simulink model "FM_V6_Zikun"  (R2022b)
settings: Solver=VariableStepAuto  StartTime=0.0  StopTime=1240
values from neighbouring files (symbols this model uses):
  A_fc = 550    [CNV.m]
  A_st = 1.1*A_fc*1E-4*n_cell*0.0012    (= 0.047553)    [CNV.m]
  A_T_rm = 0.005    [CNV.m]
  b11 = 0.005139    [CNV.m]
  b12 = 0.00326    [CNV.m]
  b2 = 350    [CNV.m]
  c1 = 10    [CNV.m]
  c3 = 2    [CNV.m]
  cc = 30    [CNV.m]
  Cd_rm = 0.0124    [CNV.m]
  Cp_air = 1005    [CNV.m]
  Cp_cl = 4180    [CNV.m]
  Cp_st = Cp_Al*1.5    (= 1350)    [CNV.m]
  F = 96485    [CNV.m]
  gamma = 1.4    [CNV.m]
  H_conv_st = 3    [CNV.m]
  i_max = 2.2    [CNV.m]
  k_ca_out = 0.2177*10^(-5)    (= 2.177e-06)    [CNV.m]
  K_sm_out = 0.3629*10^-5    (= 3.629e-06)    [CNV.m]
  kd_cp = 0.01    [CNV.m]
  kd_rm = 0    [CNV.m]
  ki_cp = 0.1    [CNV.m]
  ki_fan = -1E-5    (= -1e-05)    [CNV.m]
  ki_rm = -5E-8    (= -5e-08)    [CNV.m]
  kp_cp = 7.5    [CNV.m]
  kp_fan = -0.5    [CNV.m]
  kp_rm = -8E-7    (= -8e-07)    [CNV.m]
  M_a = 29*10^-3    (= 0.029)    [CNV.m]
  M_H2 = 2*10^-3    (= 0.002)    [CNV.m]
  m_H2_initial = P_atm*V_an/(R_H2*T_atm)    (= 0.00044494386048)    [CNV.m]
  m_H2O_initial = 0.005    [CNV.m]
  M_m_dry = 1.1    [CNV.m]
  M_N2 = 28*10^-3    (= 0.028)    [CNV.m]
  m_N2_initial = P_atm*(1-y_O2)*V_ca/(R_N2*T_atm)    (= 0.00586138039643)    [CNV.m]
  M_O2 = 32*10^-3    (= 0.032)    [CNV.m]
  m_O2_initial = P_atm*y_O2*V_ca/(R_O2*T_atm)    (= 0.00177998712422)    [CNV.m]
  m_st = n_cell*A_fc*t_m*rho_m_dry+(V_ca+V_an)*rho_Al*2.5    (= 87.4506875)    [CNV.m]
  M_v = 18*10^-3    (= 0.018)    [CNV.m]
  n_cell = 655    [CNV.m]
  P_a = P_atm*(1-L*h/T_atm)^(g*M_a/(R*L))    [CNV.m]
  P_atm = 101.25*10^3    (= 101250)    [CNV.m]
  P_ca_ref = 2.5*P_a    [CNV.m]
  phi_a = 0.1    [CNV.m]
  phi_des = 1    [CNV.m]
  R = 8.315    [CNV.m]
  R_a = 286.9    [CNV.m]
  R_H2 = 4124.3    [CNV.m]
  R_N2 = 296.8    [CNV.m]
  R_O2 = 259.8    [CNV.m]
  R_v = 461.5    [CNV.m]
  rho_a = P_a/(R_a*T_a)    [CNV.m]
  rho_H2 = 0.0899    [CNV.m]
  rho_m_dry = 0.002    [CNV.m]
  rho_N2 = 1.165    [CNV.m]
  T_a = T_atm-h*L    [CNV.m]
  T_atm = 298.15    [CNV.m]
  T_cl = 353.15    [CNV.m]
  t_m = 0.01    [CNV.m]
  T_rm = 303.15    [CNV.m]
  T_st_ref = 353.15    [CNV.m]
  V_an = n_cell*A_fc*10^(-4)*0.0005*0.3    (= 0.00540375)    [CNV.m]
  V_ca = n_cell*A_fc*10^(-4)*0.0006*0.3    (= 0.0064845)    [CNV.m]
  V_rm = 0.005    [CNV.m]
  V_sm = 0.02    [CNV.m]
  y_O2_ca_in = 0.21    [CNV.m]
libraries: fl_lib x64, nesl_utility x40, ee_lib x18, fl_ps_legacy_lib x6, SimscapeFluids_lib x5, slpidlib x4, simulink x3, batteryecm_lib x1, autolibshared x1
(part 1 of 6)
settings Model: SimulationMode=accelerator  Creator=wangz  LastModifiedBy=wangz
settings SolverCC: ZeroCrossAlgorithm=Adaptive
settings DebuggingCC: AlgebraicLoopMsg=none  IgnoredZcDiagnostic=none

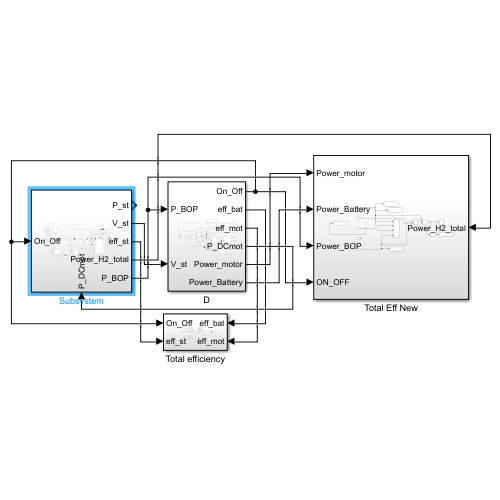
[thumbnail: Simulink's stored preview of the top-level diagram]
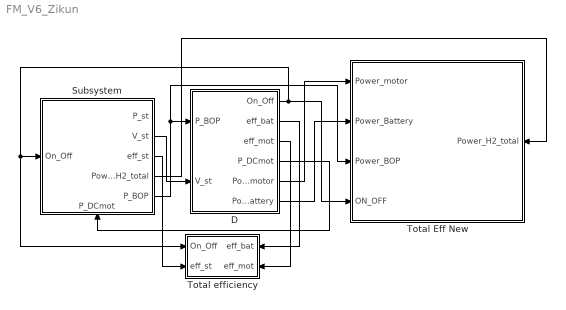
== system FM_V6_Zikun ==
  D : Subsystem
  Subsystem : Subsystem
      settings: PortSchema="{\"entries\":[{\"content\":{\"sides\":[{\"content\":{\"connectorIds\":[\"In1\"]},\"type\":\"ConnectorPlacement.EquallySpacedRectSide\",\"uuid\":\"ed2605ec-5a5c-4b25-8055-3508ff9f91b4\"},{\"content\":{\"connectorIds\":[\"Out1\",\"Out2\",\"Out3\",\"Out4\",\"Out5\"],\"side\":\"RIGHT\"},\"type\":\"ConnectorPlacement.EquallySpacedRectSide\",\"uuid\":\"d8034111-d04c-4b56-aed5-c8c9593f50d4\"},{\"content\":{\"connectorIds\":[],\"side\":\"TOP\"},\"type\":\"ConnectorPlacement.EquallySpacedRectSide\",\"uuid\":\"957209cb-ca5b-4819-85a0-7d512b0feccc\"},{\"content\":{\"connectorIds\":[\"In2\"],\"side\":\"BOTTOM\"},\"type\":\"ConnectorPlacement.EquallySpacedRectSide\",\"uuid\":\"fbb682b9-07a1-40b3-a189-215cd31ab17e\"}]},\"type\":\"ConnectorPlacement.EquallySpacedConnector\",\"uuid\":\"d905f0cd-1c81-4816-97f8-2818f3b2ae86\"}],\"packageUris\":[\"http://schema.mathworks.com/mf0/Connector/R2020b\"],\"version\":\"1.0\"}"
  Total Eff New : Subsystem
      settings: PortSchema="{\"entries\":[{\"content\":{\"sides\":[{\"content\":{\"connectorIds\":[\"In1\",\"In2\",\"In3\",\"In4\"]},\"type\":\"ConnectorPlacement.EquallySpacedRectSide\",\"uuid\":\"ccbc05d8-a6be-425d-bac9-d2d12f47e9c2\"},{\"content\":{\"connectorIds\":[\"In5\"],\"side\":\"RIGHT\"},\"type\":\"ConnectorPlacement.EquallySpacedRectSide\",\"uuid\":\"b1a7ebd3-6919-4dbb-a6bb-e13314f77759\"},{\"content\":{\"connectorIds\":[],\"side\":\"TOP\"},\"type\":\"ConnectorPlacement.EquallySpacedRectSide\",\"uuid\":\"0e0157dc-f441-4274-8930-5adc8e4ce76d\"}]},\"type\":\"ConnectorPlacement.EquallySpacedConnector\",\"uuid\":\"397d875f-74dd-4365-9efb-9b4ac1b8ecd7\"}],\"packageUris\":[\"http://schema.mathworks.com/mf0/Connector/R2020b\"],\"version\":\"1.0\"}"
  Total efficiency : Subsystem
      settings: PortSchema="{\"entries\":[{\"content\":{\"sides\":[{\"content\":{\"connectorIds\":[\"In1\",\"In2\"]},\"type\":\"ConnectorPlacement.EquallySpacedRectSide\",\"uuid\":\"73d8e2b7-5902-41f8-84e7-33ba527ac65e\"},{\"content\":{\"connectorIds\":[\"In3\",\"In4\"],\"side\":\"RIGHT\"},\"type\":\"ConnectorPlacement.EquallySpacedRectSide\",\"uuid\":\"29d9c0af-5dc9-4fa5-b074-af65dbefae33\"},{\"content\":{\"connectorIds\":[],\"side\":\"TOP\"},\"type\":\"ConnectorPlacement.EquallySpacedRectSide\",\"uuid\":\"1045b7b6-d6f6-4c04-92de-fdd7aadfc342\"}]},\"type\":\"ConnectorPlacement.EquallySpacedConnector\",\"uuid\":\"10111a07-9c9a-402f-9883-3b10a64c466d\"}],\"packageUris\":[\"http://schema.mathworks.com/mf0/Connector/R2020b\"],\"version\":\"1.0\"}"
  wires:
  Subsystem/2(V_st) -> D/2(V_st)
  D/1(On_Off) -> Total efficiency/1(On_Off), Subsystem/1(On_Off), Total Eff New/4(ON_OFF)
  Subsystem/3(eff_st) -> Total efficiency/2(eff_st)
  D/2(eff_bat) -> Total efficiency/3(eff_bat)
  D/3(eff_mot) -> Total efficiency/4(eff_mot)
  D/4(P_DCmot) -> Subsystem/2(P_DCmot)
  D/5(Power_motor) -> Total Eff New/1(Power_motor)
  D/6(Power_Battery) -> Total Eff New/2(Power_Battery)
  Subsystem/4(Power_H2_total) -> Total Eff New/5(Power_H2_total)
  Subsystem/5(P_BOP) -> Total Eff New/3(Power_BOP), D/1(P_BOP)

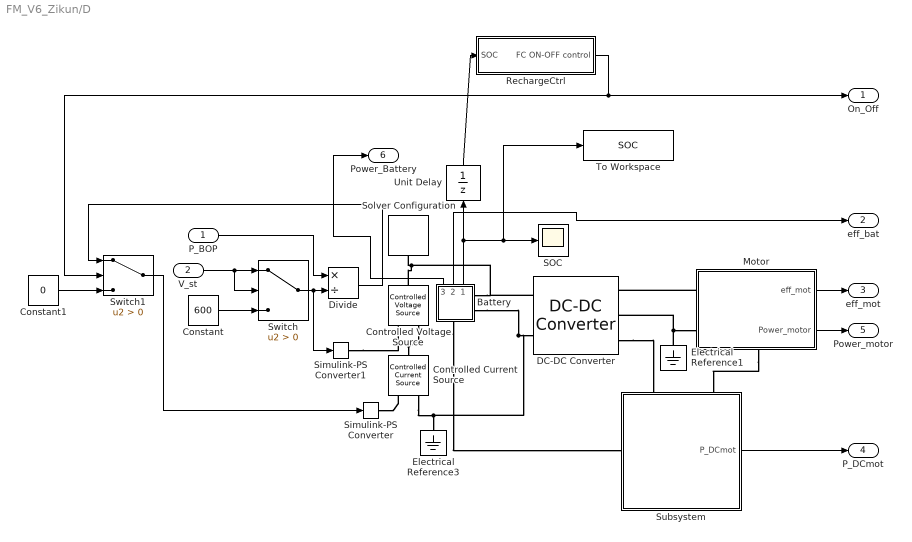
== system FM_V6_Zikun/D ==
  P_BOP : Inport
  V_st : Inport  Port=2
  Battery : Subsystem
      settings: PortSchema="{\"entries\":[{\"content\":{\"sides\":[{\"content\":{\"connectorIds\":[\"LConn1\",\"LConn2\"]},\"type\":\"ConnectorPlacement.EquallySpacedRectSide\",\"uuid\":\"97cdf077-cde5-4d24-a92d-b83c40bda79a\"},{\"content\":{\"connectorIds\":[],\"side\":\"RIGHT\"},\"type\":\"ConnectorPlacement.EquallySpacedRectSide\",\"uuid\":\"17e0717d-e8f0-41b7-b76b-51578cdfa79d\"},{\"content\":{\"connectorIds\":[\"Out1\",\"Out2\",\"Out3\"],\"side\":\"TOP\"},\"type\":\"ConnectorPlacement.EquallySpacedRectSide\",\"uuid\":\"3581f59d-6d8d-4808-a072-d33a3c8fe489\"},{\"content\":{\"connectorIds\":[\"RConn1\"],\"side\":\"BOTTOM\"},\"type\":\"ConnectorPlacement.EquallySpacedRectSide\",\"uuid\":\"b39236fb-a868-40d7-ae60-2a107db7d7ac\"}]},\"type\":\"ConnectorPlacement.EquallySpacedConnector\",\"uuid\":\"e23e8761-7535-42b0-898b-b936625f5d1f\"}],\"packageUris\":[\"http://schema.mathworks.com/mf0/Connector/R2020b\"],\"version\":\"1.0\"}"
      mask Display:
      | % Plot points to set plot range
      | color('white');plot(1.5, 2.5);plot(-1.5, -2)
      | color('black');
      | % Battery icon
      | plot([0 0], [2.5 1.3])
      | plot([0 0], [-0.6 -1.6])
      | patch([-1 1 1 -1]*0.4, [1 1 -1 -1]*0.15+0.7,[0;0;0]);
      | patch([-1 1 1 -1]*0.4, [1 1 -1 -1]*0.15-0.6,[0;0;0]);
      | patch([-1 1 1 -1]*0.8, [1 1 -1 -1]*0.15+1.3,[0;0;0]);
      | patch([-1 1 1 -1]*0.8, [1 1 -1 -1]*0.15+0.0,[0;0;0]);
  Constant : Constant  Value=600
  Constant1 : Constant  Value=0  VectorParams1D=off
  Controlled Current Source : fl_lib/Electrical/Electrical Sources/Controlled Current Source
  Controlled Voltage Source : fl_lib/Electrical/Electrical Sources/Controlled Voltage Source
  DC-DC Converter : ee_lib/Semiconductors & Converters/Converters/DC-DC Converter  Vref_option=ee.enum.converters.voltageref.internal  v_ref=600 V  P_rated=380 kW  droop_enabled=false  droop_param=ee.enum.converters.droop.value  droop=0.1 V/A  droop_percent=2  Vref_droop=10 V  reversible=ee.enum.converters.directionality.unidirectional  G_diode=1e-8 1/Ohm  P_fixed=1 W  losses_option=ee.enum.converters.lossesOption.proportionalToSquaredCurrent  eff_rated=80  tableOption=ee.enum.converters.lossTableOptionThermal.currentTemp  i_eff_vec=[-2, -1, 1, 2] A  v_eff_vec=[15, 30, 45] V  eff_vec=[66, 76, 80, 74]  eff_2D_table=[66, 66, 66; 76, 76, 76; 80, 80, 80; 74, 74, 74]  model_dynamics=ee.enum.converters.dynamics.no  tau=0.02 s  v_ini=10 V  v1_min=1 V  R1=1000 Ohm  R2=1000 Ohm  enable_fault=simscape.enum.onoff.off  fault_condition=ee.enum.faults.faultInputCondition.greaterThan  fault_threshold=0.5  T_eff_vec=[280, 300, 320] K  eff_3D_table=repmat([66; 76; 80; 74], 1, 3, 3)  thermal_mass=100 J/K  initial_temperature=T_a K
      settings: InternalSimscapePortConfiguration="{\"Bottom\":[],\"Left\":[{\"id\":\"p1\",\"label\":\"1+\",\"type\":\"foundation.electrical.electrical\"},{\"id\":\"n1\",\"label\":\"1-\",\"type\":\"foundation.electrical.electrical\"}],\"Right\":[{\"id\":\"p2\",\"label\":\"2+\",\"type\":\"foundation.electrical.electrical\"},{\"id\":\"n2\",\"label\":\"2-\",\"type\":\"foundation.electrical.electrical\"},{\"id\":\"H\",\"label\":\"H\",\"type\":\"foundation.thermal.thermal\"}],\"Top\":[]}"
  Divide : Product  Inputs=*/
  Electrical Reference1 : fl_lib/Electrical/Electrical Elements/Electrical Reference
  Electrical Reference3 : fl_lib/Electrical/Electrical Elements/Electrical Reference
  Motor : Subsystem  Tag=PublishSubsystem
      settings: PortSchema="{\"entries\":[{\"content\":{\"sides\":[{\"content\":{\"connectorIds\":[\"Out1\",\"Out2\"]},\"type\":\"ConnectorPlacement.EquallySpacedRectSide\",\"uuid\":\"9faf53df-ed0d-48a6-a829-4cc0afc935c3\"},{\"content\":{\"connectorIds\":[\"RConn1\",\"RConn2\"],\"side\":\"RIGHT\"},\"type\":\"ConnectorPlacement.EquallySpacedRectSide\",\"uuid\":\"5432dbd9-43fc-4d87-afe0-6b62fd7ab721\"},{\"content\":{\"connectorIds\":[],\"side\":\"TOP\"},\"type\":\"ConnectorPlacement.EquallySpacedRectSide\",\"uuid\":\"668ec926-dd38-4986-bab7-4e7b6e20e17b\"},{\"content\":{\"connectorIds\":[\"RConn3\"],\"side\":\"BOTTOM\"},\"type\":\"ConnectorPlacement.EquallySpacedRectSide\",\"uuid\":\"380b3fe2-26c7-41b8-98a6-53abdb207c0a\"}]},\"type\":\"ConnectorPlacement.EquallySpacedConnector\",\"uuid\":\"d6b1d22c-3806-47fa-be9f-2faf034c7b8a\"}],\"packageUris\":[\"http://schema.mathworks.com/mf0/Connector/R2020b\"],\"version\":\"1.0\"}"
      mask Display:
      | % Circle
      | plot(sin(0:0.1:2.2*pi)*0.9,cos(0:0.1:2.2*pi)*0.9);
      | 
      | % In/out
      | plot([-1.5 -0.9],[0 0]);
      | plot([1.5 0.58],[1 1]*0.65);
      | plot([1.5 0.55],-[1 1]*0.68);
      | 
      | % 'M'
      | plot([0.5 0.5],[-0.5 0.5]);
      | plot([-0.5 -0.5],[-0.5 0.5]);
      | plot([0.5 0],[0.5 -0.5]);
      | plot([-0.5 0],[0.5 -0.5]);
      | 
      | % Plot points to set plot range
      | color('white');plot(1.9,1.2);plot(-1.9,-1.2)
      | color('black');
  RechargeCtrl : Subsystem
  SOC : Scope
  Simulink-PS Converter : nesl_utility/Simulink-PS Converter  PhysicalDomain=network_engine_domain  SubClassName=ps_input  LeftPortType=input  RightPortType=output  PseudoPeriodic=off  Frequencies=[]  NoiseDistribution=none  NoiseParameters=[]  Unit=1  AffineConversion=off  FilteringAndDerivatives=provide  SimscapeFilterOrder=1  InputFilterTimeConstant=0.001  UdotUserProvided=0
  Simulink-PS Converter1 : nesl_utility/Simulink-PS Converter  PhysicalDomain=network_engine_domain  SubClassName=ps_input  LeftPortType=input  RightPortType=output  PseudoPeriodic=off  Frequencies=[]  NoiseDistribution=none  NoiseParameters=[]  Unit=1  AffineConversion=off  FilteringAndDerivatives=provide  SimscapeFilterOrder=1  InputFilterTimeConstant=0.001  UdotUserProvided=0
  Solver Configuration : nesl_utility/Solver Configuration  PhysicalDomain=network_engine_domain  SubClassName=solver  LeftPortType=input  RightPortType=generic  Tones=[]  Harmonics=[]  SimulateNoise=off  Profile=off  UseLocalSampling=off  EnableSwitchedLinearOptims=on  FrequencyDomain=off  UseCCode=off  RelTol=0.001  AbsTol=1e-06  MinStep=1e-09  ToWorkspace=off  RevertToSquareIcSolve=off  NumHomotopyIterations=100  PhasorMode=off  PhasorModeNumHarmonics=1  ConsistencySolver=NEWTON_FTOL  IndexReductionMethod=DerivativeReplacement  DoDC=off  ResidualTolerance=1e-9  ConsistencyTolSource=GLOBAL  ConsistencyAbsTol=0.001  ConsistencyRelTol=0.001  ConsistencyTolFactor=0.001  UseLocalSolver=off  LocalSolverChoice=NE_BACKWARD_EULER_ADVANCER  ResolveIndetEquations=on  FunctionEvalNumThread=1  LocalSolverSampleTime=Ts  DoFixedCost=off  MaxNonlinIter=4  MaxModeIter=2  ComputeImpulses=off  ImpulseIterations=2  LinearAlgebra=auto  LinearAlgebraNumThread=0  EquationFormulation=NE_TIME_EF  DelaysMemoryBudget=1024  AutomaticFiltering=on  FilteringTimeConstant=0.001  PartitionStorageMethod=AS_NEEDED  PartitionMemoryBudget=1024  PartitionMethod=FAST
  Subsystem : Subsystem
      settings: PortSchema="{\"entries\":[{\"content\":{\"sides\":[{\"content\":{\"connectorIds\":[\"LConn1\"]},\"type\":\"ConnectorPlacement.EquallySpacedRectSide\",\"uuid\":\"1eac062b-55d1-4813-a7c4-1da18bbd56f2\"},{\"content\":{\"connectorIds\":[\"Out1\"],\"side\":\"RIGHT\"},\"type\":\"ConnectorPlacement.EquallySpacedRectSide\",\"uuid\":\"ffbb603e-9cea-4ae8-aca3-98e58ed3fabe\"},{\"content\":{\"connectorIds\":[\"LConn2\",\"LConn3\"],\"side\":\"TOP\"},\"type\":\"ConnectorPlacement.EquallySpacedRectSide\",\"uuid\":\"c53cf24d-fc3f-43cc-9a21-a4fc5d5b89d8\"}]},\"type\":\"ConnectorPlacement.EquallySpacedConnector\",\"uuid\":\"25d1799a-311d-4a4e-a5d7-f1d0d5545db0\"}],\"packageUris\":[\"http://schema.mathworks.com/mf0/Connector/R2020b\"],\"version\":\"1.0\"}"
  Switch : Switch  Criteria=u2 > Threshold  SaturateOnIntegerOverflow=off  InputSameDT=off
  Switch1 : Switch  Criteria=u2 > Threshold  SaturateOnIntegerOverflow=off  InputSameDT=off
  To Workspace : ToWorkspace  VariableName=SOC  SaveFormat=Timeseries  SampleTime=-1
  Unit Delay : UnitDelay  SampleTime=-1  HasFrameUpgradeWarning=on
  On_Off : Outport
  eff_bat : Outport  Port=2
  eff_mot : Outport  Port=3
  P_DCmot : Outport  Port=4
  Power_motor : Outport  Port=5
  Power_Battery : Outport  Port=6
  wires:
  Battery/1(SOC) -> Unit Delay/1, To Workspace/1, SOC/1
  V_st/1 -> Switch/1, Switch/2
  Constant/1 -> Switch/3
  P_BOP/1 -> Divide/1
  Switch/1 -> Simulink-PS Converter1/1, Divide/2
  Unit Delay/1 -> RechargeCtrl/1(SOC)
  Battery/2(eff_bat) -> eff_bat/1
  Switch1/1 -> Simulink-PS Converter/1
  Constant1/1 -> Switch1/3
  Divide/1 -> Switch1/1
  RechargeCtrl/1(FC ON-OFF control) -> On_Off/1, Switch1/2
  Motor/1(eff_mot) -> eff_mot/1
  Subsystem/1(P_DCmot) -> P_DCmot/1
  Motor/2(Power_motor) -> Power_motor/1
  Battery/3(Power_Battery) -> Power_Battery/1
  connections:
  Battery/LConn2 -- DC-DC Converter/LConn2 -- Controlled Current Source/RConn2 -- Electrical Reference3/LConn1
  DC-DC Converter/LConn1 -- Battery/LConn1 -- Controlled Voltage Source/LConn1 -- Solver Configuration/RConn1
  Simulink-PS Converter/RConn1 -- Controlled Current Source/RConn1
  Motor/RConn1 -- DC-DC Converter/RConn1
  Electrical Reference1/LConn1 -- DC-DC Converter/RConn2 -- Motor/RConn2
  DC-DC Converter/RConn3 -- Subsystem/LConn2
  Battery/RConn1 -- Subsystem/LConn1
  Motor/RConn3 -- Subsystem/LConn3
  Controlled Voltage Source/RConn2 -- Controlled Current Source/LConn1
  Simulink-PS Converter1/RConn1 -- Controlled Voltage Source/RConn1

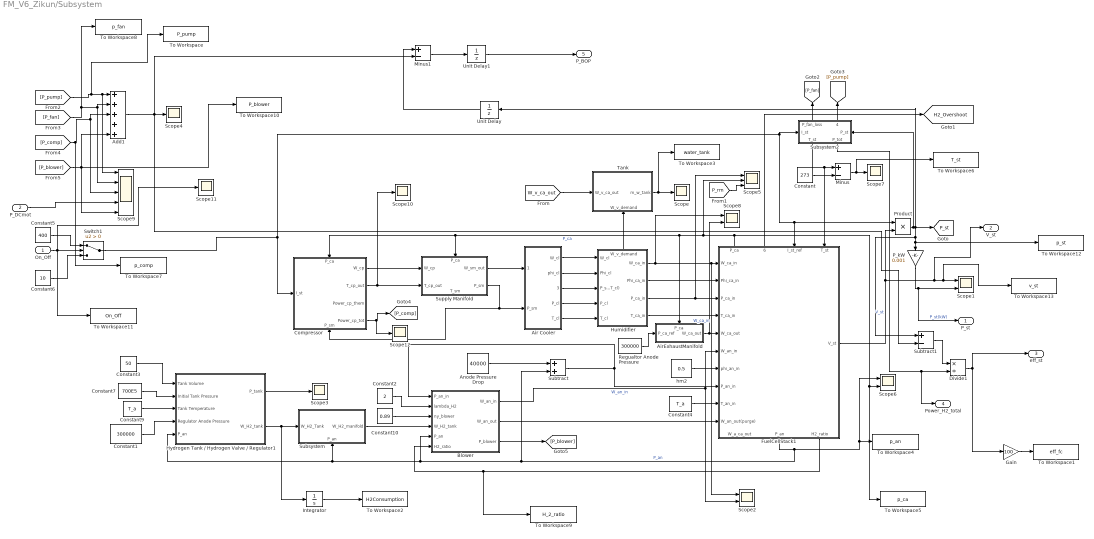
== system FM_V6_Zikun/Subsystem ==
  On_Off : Inport
  P_DCmot : Inport  Port=2
  Add1 : Sum  Inputs=+++++
  Air Cooler : Subsystem
  AirExhaustManifold : Subsystem
      settings: PortSchema="{\"entries\":[{\"content\":{\"sides\":[{\"content\":{\"connectorIds\":[\"In1\"]},\"type\":\"ConnectorPlacement.EquallySpacedRectSide\",\"uuid\":\"f4148e53-f108-416e-b09d-5cded1813cc2\"},{\"content\":{\"connectorIds\":[\"Out1\"],\"side\":\"RIGHT\"},\"type\":\"ConnectorPlacement.EquallySpacedRectSide\",\"uuid\":\"bb1370f9-51ff-4d10-85be-a4daa24eac0b\"},{\"content\":{\"connectorIds\":[\"In2\"],\"side\":\"TOP\"},\"type\":\"ConnectorPlacement.EquallySpacedRectSide\",\"uuid\":\"b6bb8738-605b-4dff-9ac0-816169ccdddf\"}]},\"type\":\"ConnectorPlacement.EquallySpacedConnector\",\"uuid\":\"dc52df26-ab55-453a-8afd-34b2548593ca\"}],\"packageUris\":[\"http://schema.mathworks.com/mf0/Connector/R2020b\"],\"version\":\"1.0\"}"
  Anode Pressure Drop : Constant  Value=40000
  Blower : Subsystem
  Compressor : Subsystem
      settings: PortSchema="{\"entries\":[{\"content\":{\"sides\":[{\"content\":{\"connectorIds\":[\"In1\"]},\"type\":\"ConnectorPlacement.EquallySpacedRectSide\",\"uuid\":\"0b68af65-198f-4122-8dac-a88f0917ed40\"},{\"content\":{\"connectorIds\":[\"Out1\",\"Out2\",\"Out3\",\"Out4\"],\"side\":\"RIGHT\"},\"type\":\"ConnectorPlacement.EquallySpacedRectSide\",\"uuid\":\"38a4b893-5b82-44e6-8bf4-e5f028da13ed\"},{\"content\":{\"connectorIds\":[\"In2\"],\"side\":\"TOP\"},\"type\":\"ConnectorPlacement.EquallySpacedRectSide\",\"uuid\":\"868a772d-c6d6-4d05-9787-210479479117\"},{\"content\":{\"connectorIds\":[\"In3\"],\"side\":\"BOTTOM\"},\"type\":\"ConnectorPlacement.EquallySpacedRectSide\",\"uuid\":\"511e7ae2-1a47-4b90-b59d-baad779358b7\"}]},\"type\":\"ConnectorPlacement.EquallySpacedConnector\",\"uuid\":\"9d0ee798-57da-47b4-8fd4-004f359c3bae\"}],\"packageUris\":[\"http://schema.mathworks.com/mf0/Connector/R2020b\"],\"version\":\"1.0\"}"
  Constant : Constant  Value=273
  Constant1 : Constant  Value=300000
  Constant10 : Constant  Value=0.89
  Constant2 : Constant  Value=2
  Constant3 : Constant  Value=50
  Constant4 : Constant  Value=T_a
  Constant5 : Constant  Value=400
  Constant6 : Constant  Value=10
  Constant7 : Constant  Value=700E5
  Constant9 : Constant  Value=T_a
  Divide1 : Product  Inputs=*/
  FuelCellStack1 : Subsystem
      settings: PortSchema="{\"entries\":[{\"content\":{\"sides\":[{\"content\":{\"connectorIds\":[\"In1\",\"In2\",\"In3\",\"In4\",\"In5\",\"In6\",\"In7\",\"In8\",\"In9\",\"In10\"]},\"type\":\"ConnectorPlacement.EquallySpacedRectSide\",\"uuid\":\"30f8b528-35d2-4863-8690-cfe5cd93b52f\"},{\"content\":{\"connectorIds\":[\"Out1\"],\"side\":\"RIGHT\"},\"type\":\"ConnectorPlacement.EquallySpacedRectSide\",\"uuid\":\"c8f65284-a774-4f7f-9711-54398f379272\"},{\"content\":{\"connectorIds\":[\"Out5\",\"Out6\",\"In11\",\"In12\"],\"side\":\"TOP\"},\"type\":\"ConnectorPlacement.EquallySpacedRectSide\",\"uuid\":\"6b67fb6e-9b2e-49bb-a93c-00120c0fdac2\"},{\"content\":{\"connectorIds\":[\"Out2\",\"Out3\",\"Out4\"],\"side\":\"BOTTOM\"},\"type\":\"ConnectorPlacement.EquallySpacedRectSide\",\"uuid\":\"be8dd292-35c4-477a-94a0-0da638b76a44\"}]},\"type\":\"ConnectorPlacement.EquallySpacedConnector\",\"uuid\":\"bdb411c7-9313-40e4-8e3b-2162bd12f23e\"}],\"packageUris\":[\"http://schema.mathworks.com/mf0/Connector/R2020b\"],\"version\":\"1.0\"}"
  Gain : Gain  Gain=100
  Humidifier : Subsystem
      settings: PortSchema="{\"entries\":[{\"content\":{\"sides\":[{\"content\":{\"connectorIds\":[\"In1\",\"In2\",\"In3\",\"In4\",\"In5\"]},\"type\":\"ConnectorPlacement.EquallySpacedRectSide\",\"uuid\":\"588083b3-912c-4b5b-b9ed-168d53ac3dd4\"},{\"content\":{\"connectorIds\":[\"Out1\",\"Out2\",\"Out3\",\"Out4\"],\"side\":\"RIGHT\"},\"type\":\"ConnectorPlacement.EquallySpacedRectSide\",\"uuid\":\"b2f7d500-3275-46d7-b9f4-632cafaed74e\"},{\"content\":{\"connectorIds\":[\"Out5\"],\"side\":\"TOP\"},\"type\":\"ConnectorPlacement.EquallySpacedRectSide\",\"uuid\":\"b2750c74-201c-41ba-a940-1f5056cf117b\"},{\"content\":{\"connectorIds\":[],\"side\":\"BOTTOM\"},\"type\":\"ConnectorPlacement.EquallySpacedRectSide\",\"uuid\":\"ef8912c5-82e4-486c-a863-02b84839332c\"}]},\"type\":\"ConnectorPlacement.EquallySpacedConnector\",\"uuid\":\"ce95aa0c-05c3-4ef9-8885-7e64e15d733d\"}],\"packageUris\":[\"http://schema.mathworks.com/mf0/Connector/R2020b\"],\"version\":\"1.0\"}"
  Hydrogen Tank / Hydrogen Valve / Regulator1 : Subsystem
  Integrator : Integrator
  Minus : Sum  Inputs=+-
  Minus1 : Sum  Inputs=+-
  P_kW : Gain  Gain=0.001
  Product : Product
  Regualtor Anode Pressure : Constant  Value=300000
  Scope{,3..4,7,10..12} (7 alike) : Scope
  Scope{1..2,6,8} (4 alike) : Scope  NumInputPorts=2
  Scope5 : Scope  NumInputPorts=3
  Scope9 : Scope  NumInputPorts=5
  Subsystem : Subsystem
      settings: PortSchema="{\"entries\":[{\"content\":{\"sides\":[{\"content\":{\"connectorIds\":[\"In1\"]},\"type\":\"ConnectorPlacement.EquallySpacedRectSide\",\"uuid\":\"215aed70-c11e-46c9-9055-ecd58b9e0011\"},{\"content\":{\"connectorIds\":[\"Out1\"],\"side\":\"RIGHT\"},\"type\":\"ConnectorPlacement.EquallySpacedRectSide\",\"uuid\":\"43785056-7026-4462-88c5-a0caec00493f\"},{\"content\":{\"connectorIds\":[],\"side\":\"TOP\"},\"type\":\"ConnectorPlacement.EquallySpacedRectSide\",\"uuid\":\"89a8e204-a418-42e7-9e12-71f1f1475410\"},{\"content\":{\"connectorIds\":[\"In2\"],\"side\":\"BOTTOM\"},\"type\":\"ConnectorPlacement.EquallySpacedRectSide\",\"uuid\":\"5978fc6c-ea0b-4ded-9f09-73f71066395c\"}]},\"type\":\"ConnectorPlacement.EquallySpacedConnector\",\"uuid\":\"0912f355-7e77-44f3-a959-38ae818581d6\"}],\"packageUris\":[\"http://schema.mathworks.com/mf0/Connector/R2020b\"],\"version\":\"1.0\"}"
  Subsystem2 : Subsystem
      settings: PortSchema="{\"entries\":[{\"content\":{\"sides\":[{\"content\":{\"connectorIds\":[\"In1\"]},\"type\":\"ConnectorPlacement.EquallySpacedRectSide\",\"uuid\":\"215aed70-c11e-46c9-9055-ecd58b9e0011\"},{\"content\":{\"connectorIds\":[\"In2\"],\"side\":\"RIGHT\"},\"type\":\"ConnectorPlacement.EquallySpacedRectSide\",\"uuid\":\"43785056-7026-4462-88c5-a0caec00493f\"},{\"content\":{\"connectorIds\":[\"Out3\",\"Out4\"],\"side\":\"TOP\"},\"type\":\"ConnectorPlacement.EquallySpacedRectSide\",\"uuid\":\"89a8e204-a418-42e7-9e12-71f1f1475410\"},{\"content\":{\"connectorIds\":[\"Out1\",\"Out2\"],\"side\":\"BOTTOM\"},\"type\":\"ConnectorPlacement.EquallySpacedRectSide\",\"uuid\":\"cb4d6ecb-2abd-4c35-ae65-20c511b8984a\"}]},\"type\":\"ConnectorPlacement.EquallySpacedConnector\",\"uuid\":\"0912f355-7e77-44f3-a959-38ae818581d6\"}],\"packageUris\":[\"http://schema.mathworks.com/mf0/Connector/R2020b\"],\"version\":\"1.0\"}"
  Subtract : Sum
  Subtract1 : Sum  Inputs=+-
  Supply Manifold : Subsystem
      settings: PortSchema="{\"entries\":[{\"content\":{\"sides\":[{\"content\":{\"connectorIds\":[\"In1\",\"In2\"]},\"type\":\"ConnectorPlacement.EquallySpacedRectSide\",\"uuid\":\"cf2033c7-28e6-43fb-8d26-233fbe9181e9\"},{\"content\":{\"connectorIds\":[\"Out1\",\"Out2\"],\"side\":\"RIGHT\"},\"type\":\"ConnectorPlacement.EquallySpacedRectSide\",\"uuid\":\"937b127f-e748-4863-bdef-8806cd909e9e\"},{\"content\":{\"connectorIds\":[\"In3\"],\"side\":\"TOP\"},\"type\":\"ConnectorPlacement.EquallySpacedRectSide\",\"uuid\":\"9bf9aeec-26a1-4af5-8d9d-99914358fc54\"},{\"content\":{\"connectorIds\":[\"Out3\"],\"side\":\"BOTTOM\"},\"type\":\"ConnectorPlacement.EquallySpacedRectSide\",\"uuid\":\"d8d253d3-4116-4650-a462-8a95da065aa3\"}]},\"type\":\"ConnectorPlacement.EquallySpacedConnector\",\"uuid\":\"a2ac6305-4b37-4082-b1f1-4dfc078c188f\"}],\"packageUris\":[\"http://schema.mathworks.com/mf0/Connector/R2020b\"],\"version\":\"1.0\"}"
  Switch1 : Switch  Criteria=u2 > Threshold  SaturateOnIntegerOverflow=off  InputSameDT=off
  Tank : Subsystem
      settings: PortSchema="{\"entries\":[{\"content\":{\"sides\":[{\"content\":{\"connectorIds\":[\"In1\"]},\"type\":\"ConnectorPlacement.EquallySpacedRectSide\",\"uuid\":\"d2c03d7e-1996-423b-976c-054c8bd88d01\"},{\"content\":{\"connectorIds\":[\"Out1\"],\"side\":\"RIGHT\"},\"type\":\"ConnectorPlacement.EquallySpacedRectSide\",\"uuid\":\"e0801423-d219-481e-9c4f-f60991e01c93\"},{\"content\":{\"connectorIds\":[],\"side\":\"TOP\"},\"type\":\"ConnectorPlacement.EquallySpacedRectSide\",\"uuid\":\"d1fd7f99-8610-48a6-8364-a1c4ea55303e\"},{\"content\":{\"connectorIds\":[\"In2\"],\"side\":\"BOTTOM\"},\"type\":\"ConnectorPlacement.EquallySpacedRectSide\",\"uuid\":\"041dad99-afaa-40e0-8f91-a09ec1f4c32c\"}]},\"type\":\"ConnectorPlacement.EquallySpacedConnector\",\"uuid\":\"2c132f22-98ae-44a0-b2c0-1870352b55d1\"}],\"packageUris\":[\"http://schema.mathworks.com/mf0/Connector/R2020b\"],\"version\":\"1.0\"}"
  To Workspace : ToWorkspace  VariableName=P_pump  SaveFormat=Timeseries  SampleTime=-1
  To Workspace1 : ToWorkspace  VariableName=eff_fc  SaveFormat=Timeseries  SampleTime=-1
  To Workspace10 : ToWorkspace  VariableName=P_blower  SaveFormat=Timeseries  SampleTime=-1
  To Workspace11 : ToWorkspace  VariableName=On_Off  SaveFormat=Timeseries  SampleTime=-1
  To Workspace12 : ToWorkspace  VariableName=p_st  SaveFormat=Timeseries  SampleTime=-1
  To Workspace13 : ToWorkspace  VariableName=v_st  SaveFormat=Timeseries  SampleTime=-1
  To Workspace2 : ToWorkspace  VariableName=H2Consumption  SaveFormat=Timeseries  SampleTime=-1
  To Workspace3 : ToWorkspace  VariableName=water_tank  SaveFormat=Timeseries  SampleTime=-1
  To Workspace4 : ToWorkspace  VariableName=p_an  SaveFormat=Timeseries  SampleTime=-1
  To Workspace5 : ToWorkspace  VariableName=p_ca  SaveFormat=Timeseries  SampleTime=-1
  To Workspace6 : ToWorkspace  VariableName=T_st  SaveFormat=Timeseries  SampleTime=-1
  To Workspace7 : ToWorkspace  VariableName=p_comp  SaveFormat=Timeseries  SampleTime=-1
  To Workspace8 : ToWorkspace  VariableName=p_fan  SaveFormat=Timeseries  SampleTime=-1
  To Workspace9 : ToWorkspace  VariableName=H_2_ratio  SaveFormat=Timeseries  SampleTime=-1
  Unit Delay : UnitDelay  SampleTime=-1  HasFrameUpgradeWarning=on
  Unit Delay1 : UnitDelay  SampleTime=-1  HasFrameUpgradeWarning=on
  hm2 : Constant  Value=0.5
  P_st : Outport
  V_st : Outport  Port=2
  eff_st : Outport  Port=3
  Power_H2_total : Outport  Port=4
  P_BOP : Outport  Port=5
  tag scope: H2_Overshoot=global, P_st=global
  wires:
  Hydrogen Tank / Hydrogen Valve / Regulator1/1(P_tank) -> Scope3/1
  hm2/1 -> FuelCellStack1/7(phi_an_in)
  Constant3/1 -> Hydrogen Tank / Hydrogen Valve / Regulator1/1(Tank Volume)
  P_kW/1 -> P_st/1, Scope1/2  "P_st(kW)"
  FuelCellStack1/5(P_ca) -> To Workspace5/1, Scope6/2, Scope5/2, Compressor/2(P_ca), Supply Manifold/3(P_ca), AirExhaustManifold/2(P_ca)  "P_ca"
  FuelCellStack1/1(V_st) -> V_st/1, To Workspace13/1, Scope1/1, Product/2  "V_st"
  Product/1 -> Subsystem2/2(P_st), Unit Delay/1, [P_st], Subtract1/1, To Workspace12/1, P_kW/1
  Air Cooler/2(phi_cl) -> Humidifier/2(Phi_cl)
  Air Cooler/3(psat_Tcl) -> Humidifier/3(P_sat(T_cl))
  AirExhaustManifold/1(W_ca_out) -> FuelCellStack1/5(W_ca_out), Scope8/2
  Humidifier/2(Phi_ca_in) -> FuelCellStack1/2(Phi_ca_in)
  Air Cooler/1(W_cl) -> Humidifier/1(W_cl)
  Constant7/1 -> Hydrogen Tank / Hydrogen Valve / Regulator1/2(Initial Tank Pressure)
  Humidifier/1(W_ca_in) -> FuelCellStack1/1(W_ca_in), Scope2/1, Scope8/1  "W_ca_in"
  Tank/1(m_w_tank) -> To Workspace3/1, Scope/1
  Air Cooler/5(T_cl) -> Humidifier/5(T_cl)
  Constant4/1 -> FuelCellStack1/9(T_an_in)
  Supply Manifold/1(W_sm_out) -> Air Cooler/1(W_sm_out)
  Air Cooler/4(P_cl) -> Humidifier/4(P_cl)
  Constant9/1 -> Hydrogen Tank / Hydrogen Valve / Regulator1/3(Tank Temperature)
  Subtract/1 -> FuelCellStack1/8(P_an_in), Blower/1(P_an_in)
  Humidifier/3(P_ca_in) -> FuelCellStack1/3(P_ca_in), Scope5/1
  Supply Manifold/2(P_sm) -> Air Cooler/2(P_sm), Compressor/3(P_sm)
  Compressor/2(T_cp_out) -> Scope10/1, Supply Manifold/2(T_cp_out)
  [P_rm] -> Scope5/3
  FuelCellStack1/3(P_an) -> To Workspace4/1, Scope6/1, Hydrogen Tank / Hydrogen Valve / Regulator1/5(P_an), Subsystem/2(P_an), Blower/5(P_an), Subtract/2  "P_an"
  Blower/3(P_blower) -> [P_blower]
  Anode Pressure Drop/1 -> Subtract/1
  FuelCellStack1/4(H2_ratio) -> To Workspace9/1, Blower/6(H2_ratio)
  Constant10/1 -> Blower/3(ny_blower)
  Constant2/1 -> Blower/2(lambda_H2)
  Compressor/1(W_cp) -> Supply Manifold/1(W_cp)
  Blower/2(W_an_out) -> FuelCellStack1/10(W_an_out(purge))
  Humidifier/5(W_v_demand) -> Tank/2(W_v_demand)
  Humidifier/4(T_ca_in) -> FuelCellStack1/4(T_ca_in)
  [W_v_ca_out] -> Tank/1(W_v_ca_out)
  Blower/1(W_an_in) -> FuelCellStack1/6(W_an_in), Scope2/2  "W_an_in"
  Regualtor Anode Pressure/1 -> AirExhaustManifold/1(P_ca_ref)
  FuelCellStack1/6(W_H2_overshoot) -> [H2_Overshoot]
  On_Off/1 -> To Workspace11/1, Scope11/1, Switch1/2
  Constant5/1 -> Switch1/1
  Subsystem2/1(T_st) -> Minus/1, FuelCellStack1/12(T_st)
  Subsystem2/3(P_fan_loss) -> [P_fan]
  Subsystem2/4(P_pump_loss) -> [P_pump]
  [P_pump] -> To Workspace/1, Scope9/1, Add1/1
  [P_fan] -> To Workspace8/1, Scope9/2, Add1/2
  [P_comp] -> To Workspace7/1, Scope9/3, Add1/3
  [P_blower] -> To Workspace10/1, Scope9/5, Add1/5
  Add1/1 -> Minus1/2, Subtract1/2, Scope4/1
  Constant1/1 -> Hydrogen Tank / Hydrogen Valve / Regulator1/4(Regulator Anode Pressure)
  Compressor/4(Power_cp_tot) -> Scope12/1, [P_comp]
  Constant6/1 -> Switch1/3
  Hydrogen Tank / Hydrogen Valve / Regulator1/2(W_H2_tank) -> Integrator/1, Subsystem/1(W_H2_Tank)
  Subsystem/1(W_H2_manifold) -> Blower/4(W_H2_tank)
  Subtract1/1 -> Divide1/1
  Subsystem2/2(P_tot) -> Power_H2_total/1, Divide1/2
  Minus/1 -> To Workspace6/1, Scope7/1
  Constant/1 -> Minus/2
  Gain/1 -> To Workspace1/1
  Divide1/1 -> Gain/1, eff_st/1
  P_DCmot/1 -> Scope9/4
  Integrator/1 -> To Workspace2/1
  Switch1/1 -> Subsystem2/1(I_st), FuelCellStack1/11(I_st_ref), Product/1, Compressor/1(I_st)
  Minus1/1 -> Unit Delay1/1
  Unit Delay/1 -> Minus1/1
  Unit Delay1/1 -> P_BOP/1

== system FM_V6_Zikun/Total Eff New ==
  Power_motor : Inport
  Power_Battery : Inport  Port=2
  Power_BOP : Inport  Port=3
  ON_OFF : Inport  Port=4
  Power_H2_total : Inport  Port=5
  Add : Sum  Inputs=+-
  Divide : Product  Inputs=*/
  Saturation : Saturate  UpperLimit=1  LowerLimit=0.05
  Scope : Scope  NumInputPorts=4
  Scope1 : Scope
  To Workspace : ToWorkspace  VariableName=power_motor  SaveFormat=Timeseries  SampleTime=-1
  To Workspace1 : ToWorkspace  VariableName=power_battery  SaveFormat=Timeseries  SampleTime=-1
  To Workspace2 : ToWorkspace  VariableName=power_H2  SaveFormat=Timeseries  SampleTime=-1
  To Workspace3 : ToWorkspace  VariableName=final_tot_eff  SaveFormat=Timeseries  SampleTime=-1
  To Workspace4 : ToWorkspace  VariableName=power_BOP  SaveFormat=Timeseries  SampleTime=-1
  wires:
  Power_motor/1 -> Divide/1, Scope/1, To Workspace/1
  Power_Battery/1 -> Add/2, To Workspace1/1, Scope/2
  Power_BOP/1 -> To Workspace4/1, Scope/3
  Power_H2_total/1 -> To Workspace2/1, Add/1, Scope/4
  Add/1 -> Divide/2
  Divide/1 -> Saturation/1, Scope1/1
  Saturation/1 -> To Workspace3/1

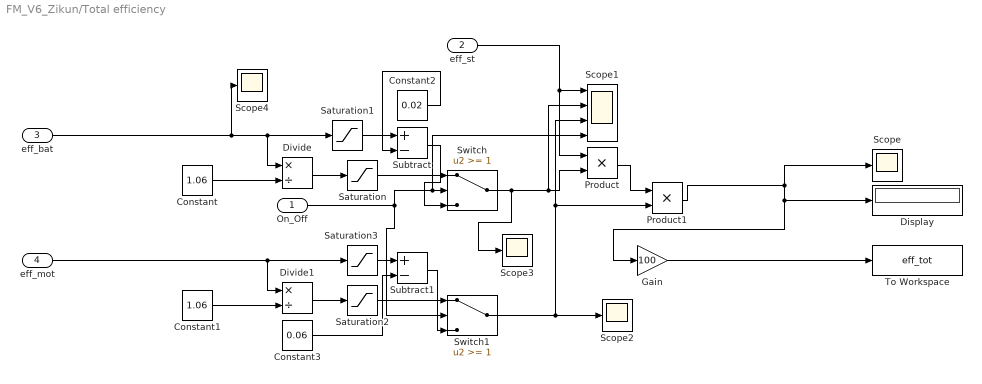
== system FM_V6_Zikun/Total efficiency ==
  On_Off : Inport
  eff_st : Inport  Port=2
  eff_bat : Inport  Port=3
  eff_mot : Inport  Port=4
  Constant : Constant  Value=1.06
  Constant1 : Constant  Value=1.06
  Constant2 : Constant  Value=0.02
  Constant3 : Constant  Value=0.06
  Display : Display
  Divide : Product  Inputs=*/
  Divide1 : Product  Inputs=*/
  Gain : Gain  Gain=100
  Product : Product
  Product1 : Product
  Saturation{,1..3} (4 alike) : Saturate  UpperLimit=1  LowerLimit=0
  Scope{,2..4} (4 alike) : Scope
  Scope1 : Scope  NumInputPorts=4
  Subtract : Sum  Inputs=+-
  Subtract1 : Sum  Inputs=+-
  Switch : Switch  Threshold=1  SaturateOnIntegerOverflow=off  InputSameDT=off
  Switch1 : Switch  Threshold=1  SaturateOnIntegerOverflow=off  InputSameDT=off
  To Workspace : ToWorkspace  VariableName=eff_tot  SaveFormat=Timeseries  SampleTime=-1
  wires:
  eff_st/1 -> Product/1, Scope1/1
  Switch/1 -> Scope3/1, Scope1/2, Product/2
  Product/1 -> Product1/1
  On_Off/1 -> Switch1/2, Scope1/4, Switch/2
  Constant/1 -> Divide/2
  eff_bat/1 -> Scope4/1, Saturation1/1, Divide/1
  Divide/1 -> Saturation/1
  Saturation/1 -> Switch/1
  Gain/1 -> To Workspace/1
  Constant1/1 -> Divide1/2
  eff_mot/1 -> Saturation3/1, Divide1/1
  Divide1/1 -> Saturation2/1
  Saturation2/1 -> Switch1/1
  Switch1/1 -> Scope2/1, Product1/2, Scope1/3
  Subtract/1 -> Switch/3
  Saturation1/1 -> Subtract/1
  Constant2/1 -> Subtract/2
  Saturation3/1 -> Subtract1/1
  Subtract1/1 -> Switch1/3
  Constant3/1 -> Subtract1/2
  Product1/1 -> Gain/1, Display/1, Scope/1

== system FM_V6_Zikun/D/Battery ==
  Battery1 : batteryecm_lib/Battery  Vnom=600 V  prm_dir=simscape.enum.battery.prm_dir.disabled  R1_dis=2 Ohm  R1_ch=2 Ohm  R1=0.001 Ohm  prm_AH=simscape.enum.battery.prm_AH.finite  AH=cc Ah  V1=540 V  AH1=cc/2 A*hr  prm_R2=1  R2=inf Ohm  prm_dyn=1  Rp1=0.005 Ohm  tau1=30 s  Rp2=0.005 Ohm  tau2=30 s  Rp3=0.005 Ohm  tau3=30 s  Rp4=0.005 Ohm  tau4=30 s  Rp5=0.005 Ohm  tau5=30 s  prm_fade=simscape.enum.battery.prm_fade.disabled  N_fade=100  AH_fade=45 hr*A  R1_fade=2.02 Ohm  R1_ch_fade=2.02 Ohm  V1_fade=10.35 V  prm_age=1  prm_age_OCV=1  OCV_age=0.9  SOC_age=60  delta_time_age_vec=[0] d  temperature_age_vec=[273] K  OCV_scaling_age=2.2134e6  OCV_offset_age=1.632e6  temp_exp_age=0.515833569 V  t_exp_age=0.75  i_specify=off  i_priority=None  i=0 A  i_nominal_specify=off  i_nominal_unit=A  i_nominal_value=1  v_specify=off  v_priority=None  v=0 V  v_nominal_specify=off  v_nominal_unit=V  v_nominal_value=1  charge_specify=on  charge_priority=High  charge=cc/2 A*hr  charge_nominal_specify=off  charge_nominal_unit=A*hr  charge_nominal_value=1  num_cycles_specify=off  num_cycles_priority=High  num_cycles=0  num_cycles_nominal_specify=off  num_cycles_nominal_unit=1  num_cycles_nominal_value=1  Tmeas=298.15 K  Tmeas_age=298.15 K  Vnom_T2=600 V  R1_T2=0.001+0.1*0.001 Ohm  R1_T2_dis=2.2 Ohm  R1_T2_ch=2.2 Ohm  V1_T2=540 V  R2_T2=2200 Ohm  Rp1_T2=0.005 Ohm  tau1_T2=30 s  Rp2_T2=0.005 Ohm  tau2_T2=30 s  Rp3_T2=0.005 Ohm  tau3_T2=30 s  Rp4_T2=0.005 Ohm  tau4_T2=30 s  Rp5_T2=0.005 Ohm  tau5_T2=30 s  Tmeas2=273.15 K  thermal_mass=89400*2 J/K  temperature_specify=on  temperature_priority=High  temperature=T_a K  temperature_nominal_specify=off  temperature_nominal_unit=K  temperature_nominal_value=1
      settings: InternalSimscapePortConfiguration="{\"Bottom\":[],\"Left\":[{\"id\":\"p\",\"label\":\"+\",\"type\":\"foundation.electrical.electrical\"},{\"id\":\"q\",\"label\":\"q\",\"type\":\"output\"}],\"Right\":[{\"id\":\"n\",\"label\":\"-\",\"type\":\"foundation.electrical.electrical\"},{\"id\":\"H\",\"label\":\"H\",\"type\":\"foundation.thermal.thermal\"}],\"Top\":[]}"
  Calculations : Subsystem
  Constant : Constant  Value=cc
  Current Sensor : fl_lib/Electrical/Electrical Sensors/Current Sensor
  Derivative : Derivative
  Divide : Product  Inputs=*/
  Multiply : Gain  Gain=3600
  PS-Simulink Converter : nesl_utility/PS-Simulink Converter  PhysicalDomain=network_engine_domain  SubClassName=ps_output  LeftPortType=input  RightPortType=output  PseudoPeriodic=off  Frequencies=[]  VectorFormat=1-D array  Unit=V  AffineConversion=off
  PS-Simulink Converter2 : nesl_utility/PS-Simulink Converter  PhysicalDomain=network_engine_domain  SubClassName=ps_output  LeftPortType=input  RightPortType=output  PseudoPeriodic=off  Frequencies=[]  VectorFormat=inherit  Unit=inherit  AffineConversion=off
  Product : Product
  Scope{,1..3} (4 alike) : Scope
  Voltage Sensor : fl_lib/Electrical/Electrical Sensors/Voltage Sensor
  + : PMIOPort  Side=Left
  - : PMIOPort  Port=2  Side=Left
  H_bat : PMIOPort  Port=3  Side=Right
  SOC : Outport
  eff_bat : Outport  Port=2
  Power_Battery : Outport  Port=3
  wires:
  PS-Simulink Converter2/1 -> Derivative/1, Scope/1, Divide/1
  Divide/1 -> SOC/1
  Constant/1 -> Multiply/1
  Multiply/1 -> Divide/2
  Calculations/1(eff_bat) -> eff_bat/1
  Derivative/1 -> Product/1, Scope1/1
  PS-Simulink Converter/1 -> Scope2/1, Product/2  "Battery power"
  Product/1 -> Scope3/1, Power_Battery/1
  connections:
  Voltage Sensor/RConn2 -- -/RConn1 -- Current Sensor/LConn1
  Current Sensor/RConn1 -- Calculations/LConn2
  Voltage Sensor/RConn1 -- PS-Simulink Converter/LConn1 -- Calculations/LConn1
  Battery1/RConn1 -- Current Sensor/RConn2
  +/RConn1 -- Battery1/LConn1 -- Voltage Sensor/LConn1
  PS-Simulink Converter2/LConn1 -- Battery1/LConn2
  H_bat/RConn1 -- Battery1/RConn2

== system FM_V6_Zikun/D/Motor ==
  Constant : Constant
  Constant1 : Constant  Value=100
  Divide : Product  Inputs=*/
  Drive Cycle Source : autolibshared/Drive Cycle Source  cycleVar=Workspace variable  wsVar=T_DRCY  fileVar=C:\Users\wangz\MATLAB Drive\TME180Project\T_DRCY.mat  tfinal="1248  seconds"  cycleRepeat=off  outAccPort=off  outGearPort=off  gearList=No gear data  t_wot1=5  xdot_woto=0  xdot_wot1=30  t_wot2=20  xdot_wot2=0  t_wotend=30  srcUnit=m/s  outUnit=m/s  srcAccUnit=m/s/s  outAccUnit=m/s^2  dt=0  aMode=1  faultOption=off  velBnd=2  velBndUnit=mph  inUnit=m/s  timeBnd=1  failOption=off  stopSim=off  maxFaultCnt=10  maxFaultTime=2  maxTotFaultTime=15  traceOption=off  dtTrace=1  traceWindow=10  lastDCname=Custom Data Set  lastOutUnit=mph  lastDT=0  lastTB=1  lastSB=2  forceCalcBound=off
  Electrical Power : Subsystem
      settings: PortSchema="{\"entries\":[{\"content\":{\"sides\":[{\"content\":{\"connectorIds\":[\"LConn1\",\"Out1\",\"LConn2\"]},\"type\":\"ConnectorPlacement.EquallySpacedRectSide\",\"uuid\":\"e9048151-2b38-4f1b-a4a4-5993aae3bd86\"},{\"content\":{\"connectorIds\":[\"RConn1\"],\"side\":\"RIGHT\"},\"type\":\"ConnectorPlacement.EquallySpacedRectSide\",\"uuid\":\"dc075957-4391-45e9-a413-1c0cb8cf4ef1\"},{\"content\":{\"connectorIds\":[],\"side\":\"TOP\"},\"type\":\"ConnectorPlacement.EquallySpacedRectSide\",\"uuid\":\"050de621-0d54-43c5-b671-a3b6dc27b776\"}]},\"type\":\"ConnectorPlacement.EquallySpacedConnector\",\"uuid\":\"7dcada06-adbf-44ac-93f3-a68dba5e4a0e\"}],\"packageUris\":[\"http://schema.mathworks.com/mf0/Connector/R2020b\"],\"version\":\"1.0\"}"
  Gain : Gain  Gain=100
  Ideal Angular Velocity Source : fl_lib/Mechanical/Mechanical Sources/Ideal Angular Velocity Source
  MRRef1 : fl_lib/Mechanical/Rotational Elements/Mechanical Rotational Reference
  MRRef2 : fl_lib/Mechanical/Rotational Elements/Mechanical Rotational Reference
  Mechanical Power : Subsystem
      settings: PortSchema="{\"entries\":[{\"content\":{\"sides\":[{\"content\":{\"connectorIds\":[\"Out1\"]},\"type\":\"ConnectorPlacement.EquallySpacedRectSide\",\"uuid\":\"9faf53df-ed0d-48a6-a829-4cc0afc935c3\"},{\"content\":{\"connectorIds\":[\"RConn1\",\"RConn2\"],\"side\":\"RIGHT\"},\"type\":\"ConnectorPlacement.EquallySpacedRectSide\",\"uuid\":\"5432dbd9-43fc-4d87-afe0-6b62fd7ab721\"},{\"content\":{\"connectorIds\":[],\"side\":\"TOP\"},\"type\":\"ConnectorPlacement.EquallySpacedRectSide\",\"uuid\":\"668ec926-dd38-4986-bab7-4e7b6e20e17b\"}]},\"type\":\"ConnectorPlacement.EquallySpacedConnector\",\"uuid\":\"d6b1d22c-3806-47fa-be9f-2faf034c7b8a\"}],\"packageUris\":[\"http://schema.mathworks.com/mf0/Connector/R2020b\"],\"version\":\"1.0\"}"
  PMSM : ee_lib/Electromechanical/Motor & Drive (System Level)  torque_speed_param=ee.enum.electromech.envelope.torque_power  overtorque_param=ee.enum.electromech.overtorque.no  T_t=[ 0.9 0.8 0.7 0 ]*500 N*m  T_t_intermittent=[.36, .32, .28, 0] N*m  T_t_2D=[.09, .09, .09; .08, .08, .08; .07, .07, .07; 0, 0, 0] N*m  T_t_intermittent_2D=[.36, .36, .36; .32, .32, .32; .28, .28, .28; 0, 0, 0] N*m  w_t=[ 0 3.75e+3 7.5e+3 8e+3 ] rpm  vdc_t=[6, 12, 24] V  torque_max=Tmax N*m  power_max=Pmax kW  torque_max_intermittent=0.4 N*m  power_max_intermittent=120 W  time_overtorque=30 s  time_recover=60 s  Tc=0.02 s  losses_param=1  eff=85  w_eff=1000 rpm  T_eff=1400 N*m  Piron=0 W  Pbase=0 W  w_eff_vec=[-8000 -4000 0 4000 8000] rpm  T_eff_vec=[0 0.03 0.06 0.09] N*m  v_eff_vec=[100, 250, 400] V  losses_mat=[1.49 1.67 2.21 3.10; 0.42 0.69 1.14 2.03; 0.06 0.24 0.78 1.68; 0.42 0.69 1.14 2.03; 1.49 1.67 2.21 3.10] W  efficiency_mat=[95 95 95 95; 95 95 95 95; 95 95 95 95; 95 95 95 95; 95 95 95 95]  losses_mat_3D=ones(5, 4, 3) W  efficiency_mat_3D=95 * ones(5, 4, 3)  Res=0 Ohm  enable_fault=simscape.enum.onoff.off  fault_condition=1  fault_threshold=0.5  J=0 kg*m^2  lam=1e-5 N*m/(rad/s)  speed0=1000 rpm  faulted_specify=off  faulted_priority=None  faulted=0  faulted_nominal_specify=off  faulted_nominal_unit=1  faulted_nominal_value=1  torqueLimitContinuous_specify=off  torqueLimitContinuous_priority=None  torqueLimitContinuous=0 N*m  torqueLimitContinuous_nominal_specify=off  torqueLimitContinuous_nominal_unit=N*m  torqueLimitContinuous_nominal_value=1  alpha=3.93e-3 1/K  Tmeas=25 degC  Tmeas2=125 degC  losses_mat_T2=[1.49, 1.74, 2.49, 3.74; .42, .67, 1.42, 2.67; .06, .31, 1.06, 2.31; .42, .67, 1.42, 2.67; 1.49, 1.74, 2.49, 3.74] W  efficiency_mat_T2=[95, 95, 95, 95; 95, 95, 95, 95; 95, 95, 95, 95; 95, 95, 95, 95; 95, 95, 95, 95]  losses_mat_3D_T2=ones(5, 4, 3) W  efficiency_mat_3D_T2=95 * ones(5, 4, 3)  thermal_mass=100 J/K  initial_temperature=T_a K
      settings: InternalSimscapePortConfiguration="{\"Bottom\":[],\"Left\":[{\"id\":\"Vp\",\"label\":\"+\",\"type\":\"foundation.electrical.electrical\"},{\"id\":\"Tr\",\"label\":\"Tr\",\"type\":\"input\"},{\"id\":\"R\",\"label\":\"R\",\"type\":\"foundation.mechanical.rotational.rotational\"}],\"Right\":[{\"id\":\"Vm\",\"label\":\"-\",\"type\":\"foundation.electrical.electrical\"},{\"id\":\"Omega\",\"label\":\"w\",\"type\":\"output\"},{\"id\":\"H\",\"label\":\"H\",\"type\":\"foundation.thermal.thermal\"},{\"id\":\"C\",\"label\":\"C\",\"type\":\"foundation.mechanical.rotational.rotational\"}],\"Top\":[]}"
  PS Product : fl_ps_legacy_lib/Legacy Physical Signals/Functions/PS Product
  PS-Simulink Converter : nesl_utility/PS-Simulink Converter  PhysicalDomain=network_engine_domain  SubClassName=ps_output  LeftPortType=input  RightPortType=output  PseudoPeriodic=off  Frequencies=[]  VectorFormat=inherit  Unit=inherit  AffineConversion=off
  PS-Simulink Converter1 : nesl_utility/PS-Simulink Converter  PhysicalDomain=network_engine_domain  SubClassName=ps_output  LeftPortType=input  RightPortType=output  PseudoPeriodic=off  Frequencies=[]  VectorFormat=inherit  Unit=inherit  AffineConversion=off
  Saturation : Saturate  UpperLimit=1  LowerLimit=0
  Scope : Scope  NumInputPorts=2
  Scope1 : Scope
  Simulink-PS Converter : nesl_utility/Simulink-PS Converter  PhysicalDomain=network_engine_domain  SubClassName=ps_input  LeftPortType=input  RightPortType=output  PseudoPeriodic=off  Frequencies=[]  NoiseDistribution=none  NoiseParameters=[]  Unit=m/s  AffineConversion=off  FilteringAndDerivatives=provide  SimscapeFilterOrder=1  InputFilterTimeConstant=0.001  UdotUserProvided=0
  Simulink-PS Converter1 : nesl_utility/Simulink-PS Converter  PhysicalDomain=network_engine_domain  SubClassName=ps_input  LeftPortType=input  RightPortType=output  PseudoPeriodic=off  Frequencies=[]  NoiseDistribution=none  NoiseParameters=[]  Unit=(N/m)/(m/s)  AffineConversion=off  FilteringAndDerivatives=provide  SimscapeFilterOrder=1  InputFilterTimeConstant=0.001  UdotUserProvided=0
  Simulink-PS Converter2 : nesl_utility/Simulink-PS Converter  PhysicalDomain=network_engine_domain  SubClassName=ps_input  LeftPortType=input  RightPortType=output  PseudoPeriodic=off  Frequencies=[]  NoiseDistribution=none  NoiseParameters=[]  Unit=1  AffineConversion=off  FilteringAndDerivatives=provide  SimscapeFilterOrder=1  InputFilterTimeConstant=0.001  UdotUserProvided=0
  Torque Sensor : fl_lib/Mechanical/Mechanical Sensors/Ideal Torque Sensor
  + : PMIOPort  Side=Right
  - : PMIOPort  Port=2  Side=Right
  H_PMSM : PMIOPort  Port=3  Side=Right
  eff_mot : Outport
  Power_motor : Outport  Port=2
  wires:
  PS-Simulink Converter/1 -> Scope/2
  Drive Cycle Source/1 -> Gain/1, Simulink-PS Converter/1, Scope/1
  Constant/1 -> Simulink-PS Converter1/1
  Constant1/1 -> Simulink-PS Converter2/1
  Electrical Power/1(Pe_motor) -> Divide/2
  Mechanical Power/1(Pm_motor) -> Divide/1
  Divide/1 -> Saturation/1
  Saturation/1 -> eff_mot/1
  PS-Simulink Converter1/1 -> Scope1/1
  Gain/1 -> Power_motor/1
  connections:
  +/RConn1 -- Electrical Power/LConn1
  PMSM/LConn1 -- Electrical Power/RConn1
  PMSM/RConn1 -- Electrical Power/LConn2 -- -/RConn1
  PMSM/LConn3 -- Torque Sensor/LConn1
  PS Product/RConn1 -- PMSM/LConn2
  Mechanical Power/RConn2 -- PS-Simulink Converter/LConn1 -- Torque Sensor/RConn2
  PMSM/RConn2 -- PS-Simulink Converter1/LConn1 -- Mechanical Power/RConn1
  Ideal Angular Velocity Source/LConn1 -- Torque Sensor/RConn1
  Simulink-PS Converter/RConn1 -- PS Product/LConn1
  Simulink-PS Converter1/RConn1 -- PS Product/LConn2
  Simulink-PS Converter2/RConn1 -- Ideal Angular Velocity Source/RConn1
  MRRef2/LConn1 -- Ideal Angular Velocity Source/RConn2
  MRRef1/LConn1 -- PMSM/RConn4
  H_PMSM/RConn1 -- PMSM/RConn3

== system FM_V6_Zikun/D/RechargeCtrl ==
  SOC : Inport
  Combinatorial Logic : CombinatorialLogic  TruthTable=[0;1;1;1;0;0;0;0]
  Compare To Constant : simulink/Logic and Bit Operations/Compare To Constant  relop=<=  const=0.415  OutDataTypeStr=boolean
  Compare To Constant1 : simulink/Logic and Bit Operations/Compare To Constant  relop=>=  const=0.585  OutDataTypeStr=boolean
  Compare To Zero : simulink/Logic and Bit Operations/Compare To Zero  relop=>  OutDataTypeStr=boolean
  Memory : Memory
  Mux1 : Mux  Inputs=3
  Scope : Scope
  FC ON-OFF control : Outport
  wires:
  Compare To Constant/1 -> Mux1/2
  Compare To Constant1/1 -> Mux1/1
  Mux1/1 -> Combinatorial Logic/1
  Compare To Zero/1 -> Mux1/3
  SOC/1 -> Compare To Constant/1, Compare To Constant1/1
  Combinatorial Logic/1 -> Memory/1, Scope/1, FC ON-OFF control/1
  Memory/1 -> Compare To Zero/1
